simulink model "Airys_Equation"  (R2024b)
settings: Solver=VariableStepAuto  StartTime=0.0  StopTime=2  RelTol=1e-3
settings Model: Creator=user  LastModifiedBy=user

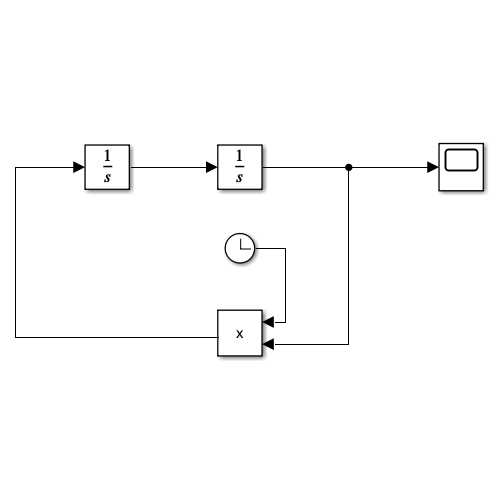
[thumbnail: Simulink's stored preview of the top-level diagram]
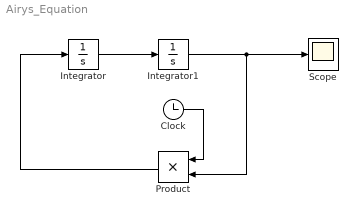
== system Airys_Equation ==
  Clock : Clock
  Integrator : Integrator  InitialCondition=1
  Integrator1 : Integrator  InitialCondition=1
  Product : Product
  Scope : Scope
  wires:
  Integrator/1 -> Integrator1/1
  Clock/1 -> Product/1
  Integrator1/1 -> Scope/1, Product/2
  Product/1 -> Integrator/1
